simulink model "simulink_multirotor_v3_taimoor"  (R2021b)
settings: Solver=VariableStepAuto  StartTime=0.0  StopTime=10  RelTol=1e-3
libraries: slpidlib x6
settings Model: Creator=five  LastModifiedBy=Muham
settings SolverCC: AlgebraicLoopSolver=TrustRegion
settings DebuggingCC: SFMachineParentedDataDiag=warning

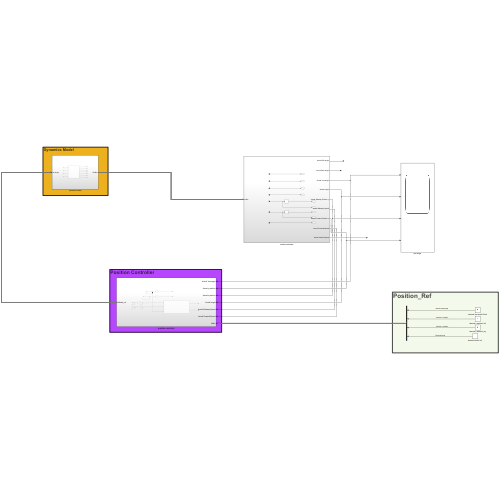
[thumbnail: Simulink's stored preview of the top-level diagram]
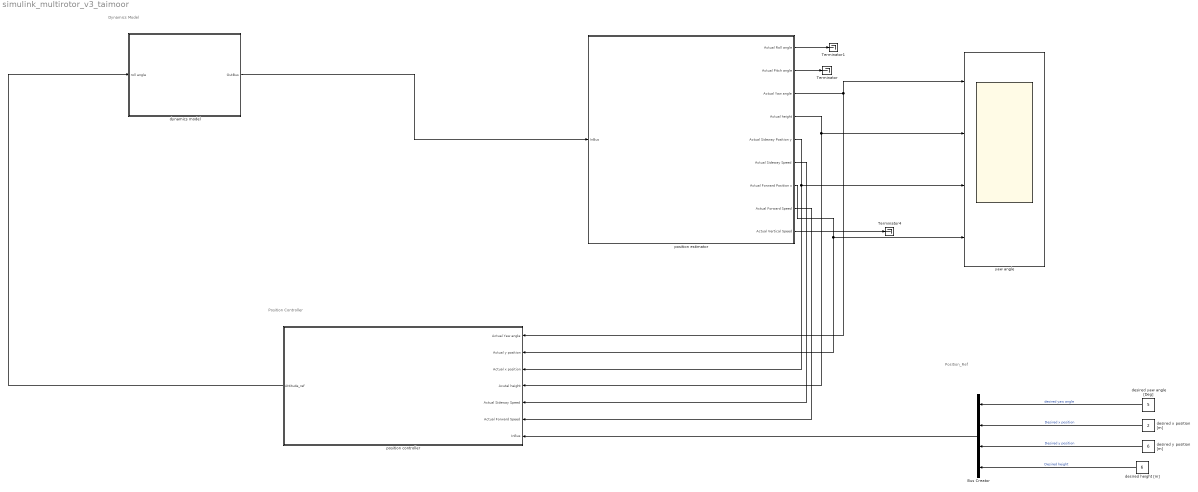
== system simulink_multirotor_v3_taimoor ==
  note: Dynamics Model
  note: Position Controller
  note: Position_Ref
  Bus Creator : BusCreator  Inputs=4
  Terminator : Terminator
  Terminator1 : Terminator
  Terminator4 : Terminator
  desired height [m] : Constant  Value=6
  desired x position [m] : Constant  Value=2
  desired y position [m] : Constant  Value=6
  desired yaw angle [Deg] : Constant  Value=5
  dynamics model : Subsystem
  position controller : Subsystem
  position estimator : Subsystem
  yaw angle : Scope  NumInputPorts=4
  wires:
  position estimator/4(Actual height) -> yaw angle/2, position controller/4(Acutal height)
  position estimator/7(Actual Forward Position x) -> position controller/2(Actual y position), yaw angle/4
  position estimator/5(Actual Sideway Position y) -> yaw angle/3, position controller/3(Actual x position)
  position estimator/3(Actual Yaw angle) -> yaw angle/1, position controller/1(Actual Yaw angle)
  position estimator/9(Actual Vertical Speed) -> Terminator4/1
  position estimator/8(Actual Forward Speed) -> position controller/6(Actual Forward Speed)
  position estimator/6(Actual Sideway Speed) -> position controller/5(Actual Sideway Speed)
  position estimator/2(Actual Pitch angle) -> Terminator/1
  position estimator/1(Actual Roll angle) -> Terminator1/1
  desired yaw angle [Deg]/1 -> Bus Creator/1  "desired yaw angle"
  desired x position [m]/1 -> Bus Creator/2  "Desired x position"
  desired y position [m]/1 -> Bus Creator/3  "Desired y position"
  desired height [m]/1 -> Bus Creator/4  "Desired height"
  Bus Creator/1 -> position controller/7(InBus)
  position controller/1(Attitude_ref) -> dynamics model/1(roll angle)
  dynamics model/1(OutBus) -> position estimator/1(InBus)

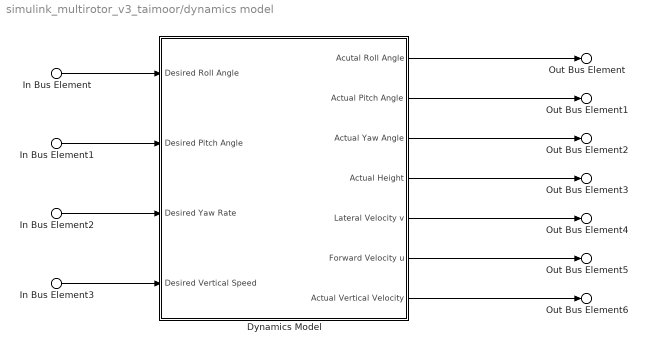
== system simulink_multirotor_v3_taimoor/dynamics model ==
  In Bus Element : Inport  PortName=roll angle  Element=desired roll angle
  In Bus Element1 : Inport  PortName=roll angle  Element=desired pitch angle
  In Bus Element2 : Inport  PortName=roll angle  Element=desired yaw rate
  In Bus Element3 : Inport  PortName=roll angle  Element=desired vertical speed
  Dynamics Model : Subsystem
  Out Bus Element : Outport  PortName=OutBus  Element=Actual Roll Angle
  Out Bus Element1 : Outport  PortName=OutBus  Element=Acutal Ptich Angle
  Out Bus Element2 : Outport  PortName=OutBus  Element=Actual Yaw Angle
  Out Bus Element3 : Outport  PortName=OutBus  Element=Actual Height
  Out Bus Element4 : Outport  PortName=OutBus  Element=Actual Sideway Speed
  Out Bus Element5 : Outport  PortName=OutBus  Element=Actual Forward Speed
  Out Bus Element6 : Outport  PortName=OutBus  Element=Actual Vertical Speed
  wires:
  In Bus Element/1 -> Dynamics Model/1(Desired Roll Angle)
  In Bus Element1/1 -> Dynamics Model/2(Desired Pitch Angle)
  In Bus Element2/1 -> Dynamics Model/3(Desired Yaw Rate)
  In Bus Element3/1 -> Dynamics Model/4(Desired Vertical Speed)
  Dynamics Model/6(Forward Velocity u) -> Out Bus Element5/1
  Dynamics Model/5(Lateral Velocity v) -> Out Bus Element4/1
  Dynamics Model/4(Actual Height) -> Out Bus Element3/1
  Dynamics Model/3(Actual Yaw Angle) -> Out Bus Element2/1
  Dynamics Model/2(Actual Pitch Angle) -> Out Bus Element1/1
  Dynamics Model/1(Acutal Roll Angle) -> Out Bus Element/1
  Dynamics Model/7(Actual Vertical Velocity) -> Out Bus Element6/1

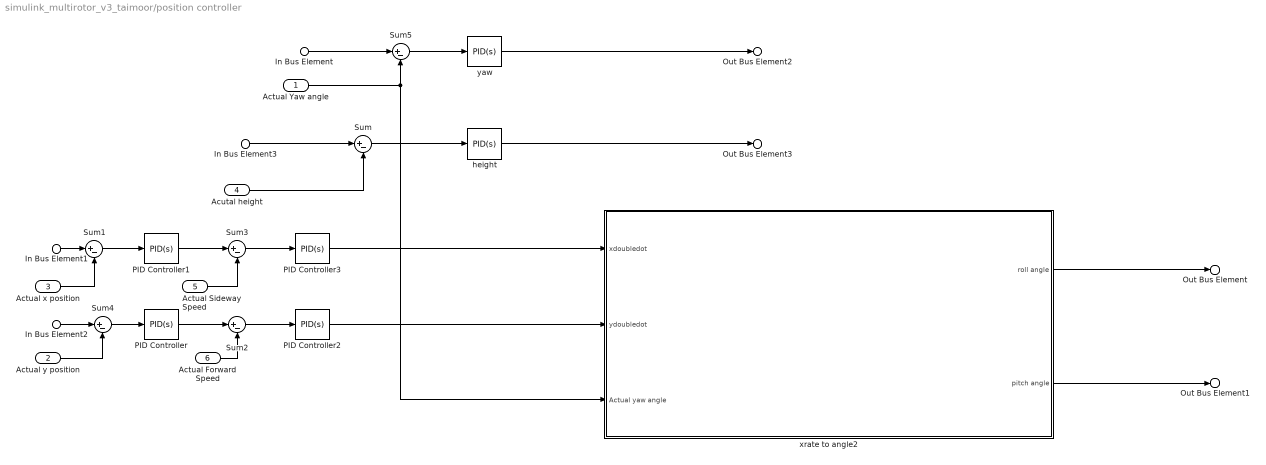
== system simulink_multirotor_v3_taimoor/position controller ==
  Actual Yaw angle : Inport
  Actual y position : Inport  Port=2
  Actual x position : Inport  Port=3
  Acutal height : Inport  Port=4
  Actual Sideway Speed : Inport  Port=5
  Actual Forward Speed : Inport  Port=6
  In Bus Element : Inport  Port=7  PortName=InBus  Element=desired yaw angle
  In Bus Element1 : Inport  Port=7  PortName=InBus  Element=Desired x position
  In Bus Element2 : Inport  Port=7  PortName=InBus  Element=Desired y position
  In Bus Element3 : Inport  Port=7  PortName=InBus  Element=Desired height
  PID Controller : slpidlib/PID Controller  Controller=PID  Form=Parallel  TimeDomain=Continuous-time  UseExternalTs=off  SampleTime=-1  IntegratorMethod=Forward Euler  FilterMethod=Forward Euler  ControllerParametersSource=internal  P=3  I=0  D=4  UseFilter=on  N=100  TunerSelectOption=Transfer Function Based (PID Tuner App)  InitialConditionSource=internal  InitialConditionForIntegrator=0  InitialConditionForFilter=0  DifferentiatorICPrevScaledInput=0  ExternalReset=none  TrackingMode=off  Kt=1  LimitOutput=off  SatLimitsSource=internal  UpperSaturationLimit=inf  LowerSaturationLimit=-inf  LinearizeAsGain=on  AntiWindupMode=none  Kb=1  POutMin=[]  POutMax=[]  IOutMin=[]  IOutMax=[]  DOutMin=[]  DOutMax=[]  NOutMin=[]  NOutMax=[]  SumOutMin=[]  SumOutMax=[]  SaturationOutMin=[]  SaturationOutMax=[]  PParamMin=[]  PParamMax=[]  IParamMin=[]  IParamMax=[]  DParamMin=[]  DParamMax=[]  NParamMin=[]  NParamMax=[]  KbParamMin=[]  KbParamMax=[]  KtParamMin=[]  KtParamMax=[]  KbOutMin=[]  KbOutMax=[]  KtOutMin=[]  KtOutMax=[]  IntegratorOutMin=[]  IntegratorOutMax=[]  FilterOutMin=[]  FilterOutMax=[]  SumI1OutMin=[]  SumI1OutMax=[]  SumI2OutMin=[]  SumI2OutMax=[]  SumI3OutMin=[]  SumI3OutMax=[]  SumI4OutMin=[]  SumI4OutMax=[]  SumDOutMin=[]  SumDOutMax=[]  DifferentiatorOutMin=[]  DifferentiatorOutMax=[]  FilterDiffOutCoefMin=[]  FilterDiffOutCoefMax=[]  ReciprocalOutMin=[]  ReciprocalOutMax=[]  SumDenOutMin=[]  SumDenOutMax=[]  SumNumOutMin=[]  SumNumOutMax=[]  DivideOutMin=[]  DivideOutMax=[]  UdiffTsProdOutMin=[]  UdiffTsProdOutMax=[]  NTsProdOutMin=[]  NTsProdOutMax=[]  UintegralTsProdOutMin=[]  UintegralTsProdOutMax=[]  UngainTsProdOutMin=[]  UngainTsProdOutMax=[]  IntegratorContinuousStateAttributes=''  IntegratorStateMustResolveToSignalObject=off  IntegratorRTWStateStorageClass=Auto  FilterContinuousStateAttributes=''  FilterStateMustResolveToSignalObject=off  FilterRTWStateStorageClass=Auto  ParallelPVariant=InternalParameters  IdealPVariant=Disabled  IVariant=InternalParameters  DVariant=InternalParameters  IntegratorVariant=Continuous  SatVariant=Disabled  AWVariant=Passthrough  PCopyVariant=Disabled  TRVariant=Disabled  FdbkBlocksVariant=Forward  IdealPFdbkVariant=Disabled  SatFdbkVariant=Disabled  DerivativeFilterVariant=ContFilter  NVariant=InternalParameters  NCopyVariant=Disabled  FilterICVariant=InternalICsFilter  IntegratorICVariant=InternalICs  ExternalResetVariant=Disabled  TRSumVariant=Passthrough  SumFdbkVariant=Disabled  SumVariant=Sum_PID  TsampFilterVariant=InternalTs  TsampNgainVariant=Passthrough  TsampIntegralVariant=Passthrough  ExternalSaturationOutDataTypeStr=Inherit: Same as second input
  PID Controller1 : slpidlib/PID Controller  Controller=PID  Form=Parallel  TimeDomain=Continuous-time  UseExternalTs=off  SampleTime=-1  IntegratorMethod=Forward Euler  FilterMethod=Forward Euler  ControllerParametersSource=internal  P=3  I=0  D=1  UseFilter=on  N=100  TunerSelectOption=Transfer Function Based (PID Tuner App)  InitialConditionSource=internal  InitialConditionForIntegrator=0  InitialConditionForFilter=0  DifferentiatorICPrevScaledInput=0  ExternalReset=none  TrackingMode=off  Kt=1  LimitOutput=off  SatLimitsSource=internal  UpperSaturationLimit=inf  LowerSaturationLimit=-inf  LinearizeAsGain=on  AntiWindupMode=none  Kb=1  POutMin=[]  POutMax=[]  IOutMin=[]  IOutMax=[]  DOutMin=[]  DOutMax=[]  NOutMin=[]  NOutMax=[]  SumOutMin=[]  SumOutMax=[]  SaturationOutMin=[]  SaturationOutMax=[]  PParamMin=[]  PParamMax=[]  IParamMin=[]  IParamMax=[]  DParamMin=[]  DParamMax=[]  NParamMin=[]  NParamMax=[]  KbParamMin=[]  KbParamMax=[]  KtParamMin=[]  KtParamMax=[]  KbOutMin=[]  KbOutMax=[]  KtOutMin=[]  KtOutMax=[]  IntegratorOutMin=[]  IntegratorOutMax=[]  FilterOutMin=[]  FilterOutMax=[]  SumI1OutMin=[]  SumI1OutMax=[]  SumI2OutMin=[]  SumI2OutMax=[]  SumI3OutMin=[]  SumI3OutMax=[]  SumI4OutMin=[]  SumI4OutMax=[]  SumDOutMin=[]  SumDOutMax=[]  DifferentiatorOutMin=[]  DifferentiatorOutMax=[]  FilterDiffOutCoefMin=[]  FilterDiffOutCoefMax=[]  ReciprocalOutMin=[]  ReciprocalOutMax=[]  SumDenOutMin=[]  SumDenOutMax=[]  SumNumOutMin=[]  SumNumOutMax=[]  DivideOutMin=[]  DivideOutMax=[]  UdiffTsProdOutMin=[]  UdiffTsProdOutMax=[]  NTsProdOutMin=[]  NTsProdOutMax=[]  UintegralTsProdOutMin=[]  UintegralTsProdOutMax=[]  UngainTsProdOutMin=[]  UngainTsProdOutMax=[]  IntegratorContinuousStateAttributes=''  IntegratorStateMustResolveToSignalObject=off  IntegratorRTWStateStorageClass=Auto  FilterContinuousStateAttributes=''  FilterStateMustResolveToSignalObject=off  FilterRTWStateStorageClass=Auto  ParallelPVariant=InternalParameters  IdealPVariant=Disabled  IVariant=InternalParameters  DVariant=InternalParameters  IntegratorVariant=Continuous  SatVariant=Disabled  AWVariant=Passthrough  PCopyVariant=Disabled  TRVariant=Disabled  FdbkBlocksVariant=Forward  IdealPFdbkVariant=Disabled  SatFdbkVariant=Disabled  DerivativeFilterVariant=ContFilter  NVariant=InternalParameters  NCopyVariant=Disabled  FilterICVariant=InternalICsFilter  IntegratorICVariant=InternalICs  ExternalResetVariant=Disabled  TRSumVariant=Passthrough  SumFdbkVariant=Disabled  SumVariant=Sum_PID  TsampFilterVariant=InternalTs  TsampNgainVariant=Passthrough  TsampIntegralVariant=Passthrough  ExternalSaturationOutDataTypeStr=Inherit: Same as second input
  PID Controller2 : slpidlib/PID Controller  Controller=PID  Form=Parallel  TimeDomain=Continuous-time  UseExternalTs=off  SampleTime=-1  IntegratorMethod=Forward Euler  FilterMethod=Forward Euler  ControllerParametersSource=internal  P=10  I=5  D=2.5  UseFilter=on  N=100  TunerSelectOption=Transfer Function Based (PID Tuner App)  InitialConditionSource=internal  InitialConditionForIntegrator=0  InitialConditionForFilter=0  DifferentiatorICPrevScaledInput=0  ExternalReset=none  TrackingMode=off  Kt=1  LimitOutput=off  SatLimitsSource=internal  UpperSaturationLimit=inf  LowerSaturationLimit=-inf  LinearizeAsGain=on  AntiWindupMode=none  Kb=1  POutMin=[]  POutMax=[]  IOutMin=[]  IOutMax=[]  DOutMin=[]  DOutMax=[]  NOutMin=[]  NOutMax=[]  SumOutMin=[]  SumOutMax=[]  SaturationOutMin=[]  SaturationOutMax=[]  PParamMin=[]  PParamMax=[]  IParamMin=[]  IParamMax=[]  DParamMin=[]  DParamMax=[]  NParamMin=[]  NParamMax=[]  KbParamMin=[]  KbParamMax=[]  KtParamMin=[]  KtParamMax=[]  KbOutMin=[]  KbOutMax=[]  KtOutMin=[]  KtOutMax=[]  IntegratorOutMin=[]  IntegratorOutMax=[]  FilterOutMin=[]  FilterOutMax=[]  SumI1OutMin=[]  SumI1OutMax=[]  SumI2OutMin=[]  SumI2OutMax=[]  SumI3OutMin=[]  SumI3OutMax=[]  SumI4OutMin=[]  SumI4OutMax=[]  SumDOutMin=[]  SumDOutMax=[]  DifferentiatorOutMin=[]  DifferentiatorOutMax=[]  FilterDiffOutCoefMin=[]  FilterDiffOutCoefMax=[]  ReciprocalOutMin=[]  ReciprocalOutMax=[]  SumDenOutMin=[]  SumDenOutMax=[]  SumNumOutMin=[]  SumNumOutMax=[]  DivideOutMin=[]  DivideOutMax=[]  UdiffTsProdOutMin=[]  UdiffTsProdOutMax=[]  NTsProdOutMin=[]  NTsProdOutMax=[]  UintegralTsProdOutMin=[]  UintegralTsProdOutMax=[]  UngainTsProdOutMin=[]  UngainTsProdOutMax=[]  IntegratorContinuousStateAttributes=''  IntegratorStateMustResolveToSignalObject=off  IntegratorRTWStateStorageClass=Auto  FilterContinuousStateAttributes=''  FilterStateMustResolveToSignalObject=off  FilterRTWStateStorageClass=Auto  ParallelPVariant=InternalParameters  IdealPVariant=Disabled  IVariant=InternalParameters  DVariant=InternalParameters  IntegratorVariant=Continuous  SatVariant=Disabled  AWVariant=Passthrough  PCopyVariant=Disabled  TRVariant=Disabled  FdbkBlocksVariant=Forward  IdealPFdbkVariant=Disabled  SatFdbkVariant=Disabled  DerivativeFilterVariant=ContFilter  NVariant=InternalParameters  NCopyVariant=Disabled  FilterICVariant=InternalICsFilter  IntegratorICVariant=InternalICs  ExternalResetVariant=Disabled  TRSumVariant=Passthrough  SumFdbkVariant=Disabled  SumVariant=Sum_PID  TsampFilterVariant=InternalTs  TsampNgainVariant=Passthrough  TsampIntegralVariant=Passthrough  ExternalSaturationOutDataTypeStr=Inherit: Same as second input
  PID Controller3 : slpidlib/PID Controller  Controller=PID  Form=Parallel  TimeDomain=Continuous-time  UseExternalTs=off  SampleTime=-1  IntegratorMethod=Forward Euler  FilterMethod=Forward Euler  ControllerParametersSource=internal  P=10  I=5  D=2.5  UseFilter=on  N=100  TunerSelectOption=Transfer Function Based (PID Tuner App)  InitialConditionSource=internal  InitialConditionForIntegrator=0  InitialConditionForFilter=0  DifferentiatorICPrevScaledInput=0  ExternalReset=none  TrackingMode=off  Kt=1  LimitOutput=off  SatLimitsSource=internal  UpperSaturationLimit=inf  LowerSaturationLimit=-inf  LinearizeAsGain=on  AntiWindupMode=none  Kb=1  POutMin=[]  POutMax=[]  IOutMin=[]  IOutMax=[]  DOutMin=[]  DOutMax=[]  NOutMin=[]  NOutMax=[]  SumOutMin=[]  SumOutMax=[]  SaturationOutMin=[]  SaturationOutMax=[]  PParamMin=[]  PParamMax=[]  IParamMin=[]  IParamMax=[]  DParamMin=[]  DParamMax=[]  NParamMin=[]  NParamMax=[]  KbParamMin=[]  KbParamMax=[]  KtParamMin=[]  KtParamMax=[]  KbOutMin=[]  KbOutMax=[]  KtOutMin=[]  KtOutMax=[]  IntegratorOutMin=[]  IntegratorOutMax=[]  FilterOutMin=[]  FilterOutMax=[]  SumI1OutMin=[]  SumI1OutMax=[]  SumI2OutMin=[]  SumI2OutMax=[]  SumI3OutMin=[]  SumI3OutMax=[]  SumI4OutMin=[]  SumI4OutMax=[]  SumDOutMin=[]  SumDOutMax=[]  DifferentiatorOutMin=[]  DifferentiatorOutMax=[]  FilterDiffOutCoefMin=[]  FilterDiffOutCoefMax=[]  ReciprocalOutMin=[]  ReciprocalOutMax=[]  SumDenOutMin=[]  SumDenOutMax=[]  SumNumOutMin=[]  SumNumOutMax=[]  DivideOutMin=[]  DivideOutMax=[]  UdiffTsProdOutMin=[]  UdiffTsProdOutMax=[]  NTsProdOutMin=[]  NTsProdOutMax=[]  UintegralTsProdOutMin=[]  UintegralTsProdOutMax=[]  UngainTsProdOutMin=[]  UngainTsProdOutMax=[]  IntegratorContinuousStateAttributes=''  IntegratorStateMustResolveToSignalObject=off  IntegratorRTWStateStorageClass=Auto  FilterContinuousStateAttributes=''  FilterStateMustResolveToSignalObject=off  FilterRTWStateStorageClass=Auto  ParallelPVariant=InternalParameters  IdealPVariant=Disabled  IVariant=InternalParameters  DVariant=InternalParameters  IntegratorVariant=Continuous  SatVariant=Disabled  AWVariant=Passthrough  PCopyVariant=Disabled  TRVariant=Disabled  FdbkBlocksVariant=Forward  IdealPFdbkVariant=Disabled  SatFdbkVariant=Disabled  DerivativeFilterVariant=ContFilter  NVariant=InternalParameters  NCopyVariant=Disabled  FilterICVariant=InternalICsFilter  IntegratorICVariant=InternalICs  ExternalResetVariant=Disabled  TRSumVariant=Passthrough  SumFdbkVariant=Disabled  SumVariant=Sum_PID  TsampFilterVariant=InternalTs  TsampNgainVariant=Passthrough  TsampIntegralVariant=Passthrough  ExternalSaturationOutDataTypeStr=Inherit: Same as second input
  Sum{,1..5} (6 alike) : Sum  Inputs=|+-
  height : slpidlib/PID Controller  Controller=PID  Form=Parallel  TimeDomain=Continuous-time  UseExternalTs=off  SampleTime=-1  IntegratorMethod=Forward Euler  FilterMethod=Forward Euler  ControllerParametersSource=internal  P=1  I=0  D=4  UseFilter=on  N=100  TunerSelectOption=Transfer Function Based (PID Tuner App)  InitialConditionSource=internal  InitialConditionForIntegrator=0  InitialConditionForFilter=0  DifferentiatorICPrevScaledInput=0  ExternalReset=none  TrackingMode=off  Kt=1  LimitOutput=off  SatLimitsSource=internal  UpperSaturationLimit=inf  LowerSaturationLimit=-inf  LinearizeAsGain=on  AntiWindupMode=none  Kb=1  POutMin=[]  POutMax=[]  IOutMin=[]  IOutMax=[]  DOutMin=[]  DOutMax=[]  NOutMin=[]  NOutMax=[]  SumOutMin=[]  SumOutMax=[]  SaturationOutMin=[]  SaturationOutMax=[]  PParamMin=[]  PParamMax=[]  IParamMin=[]  IParamMax=[]  DParamMin=[]  DParamMax=[]  NParamMin=[]  NParamMax=[]  KbParamMin=[]  KbParamMax=[]  KtParamMin=[]  KtParamMax=[]  KbOutMin=[]  KbOutMax=[]  KtOutMin=[]  KtOutMax=[]  IntegratorOutMin=[]  IntegratorOutMax=[]  FilterOutMin=[]  FilterOutMax=[]  SumI1OutMin=[]  SumI1OutMax=[]  SumI2OutMin=[]  SumI2OutMax=[]  SumI3OutMin=[]  SumI3OutMax=[]  SumI4OutMin=[]  SumI4OutMax=[]  SumDOutMin=[]  SumDOutMax=[]  DifferentiatorOutMin=[]  DifferentiatorOutMax=[]  FilterDiffOutCoefMin=[]  FilterDiffOutCoefMax=[]  ReciprocalOutMin=[]  ReciprocalOutMax=[]  SumDenOutMin=[]  SumDenOutMax=[]  SumNumOutMin=[]  SumNumOutMax=[]  DivideOutMin=[]  DivideOutMax=[]  UdiffTsProdOutMin=[]  UdiffTsProdOutMax=[]  NTsProdOutMin=[]  NTsProdOutMax=[]  UintegralTsProdOutMin=[]  UintegralTsProdOutMax=[]  UngainTsProdOutMin=[]  UngainTsProdOutMax=[]  IntegratorContinuousStateAttributes=''  IntegratorStateMustResolveToSignalObject=off  IntegratorRTWStateStorageClass=Auto  FilterContinuousStateAttributes=''  FilterStateMustResolveToSignalObject=off  FilterRTWStateStorageClass=Auto  ParallelPVariant=InternalParameters  IdealPVariant=Disabled  IVariant=InternalParameters  DVariant=InternalParameters  IntegratorVariant=Continuous  SatVariant=Disabled  AWVariant=Passthrough  PCopyVariant=Disabled  TRVariant=Disabled  FdbkBlocksVariant=Forward  IdealPFdbkVariant=Disabled  SatFdbkVariant=Disabled  DerivativeFilterVariant=ContFilter  NVariant=InternalParameters  NCopyVariant=Disabled  FilterICVariant=InternalICsFilter  IntegratorICVariant=InternalICs  ExternalResetVariant=Disabled  TRSumVariant=Passthrough  SumFdbkVariant=Disabled  SumVariant=Sum_PID  TsampFilterVariant=InternalTs  TsampNgainVariant=Passthrough  TsampIntegralVariant=Passthrough  ExternalSaturationOutDataTypeStr=Inherit: Same as second input
  xrate to angle2 : Subsystem
  yaw : slpidlib/PID Controller  Controller=PID  Form=Parallel  TimeDomain=Continuous-time  UseExternalTs=off  SampleTime=-1  IntegratorMethod=Forward Euler  FilterMethod=Forward Euler  ControllerParametersSource=internal  P=50  I=10  D=2.5  UseFilter=on  N=100  TunerSelectOption=Transfer Function Based (PID Tuner App)  InitialConditionSource=internal  InitialConditionForIntegrator=0  InitialConditionForFilter=0  DifferentiatorICPrevScaledInput=0  ExternalReset=none  TrackingMode=off  Kt=1  LimitOutput=off  SatLimitsSource=internal  UpperSaturationLimit=inf  LowerSaturationLimit=-inf  LinearizeAsGain=on  AntiWindupMode=none  Kb=1  POutMin=[]  POutMax=[]  IOutMin=[]  IOutMax=[]  DOutMin=[]  DOutMax=[]  NOutMin=[]  NOutMax=[]  SumOutMin=[]  SumOutMax=[]  SaturationOutMin=[]  SaturationOutMax=[]  PParamMin=[]  PParamMax=[]  IParamMin=[]  IParamMax=[]  DParamMin=[]  DParamMax=[]  NParamMin=[]  NParamMax=[]  KbParamMin=[]  KbParamMax=[]  KtParamMin=[]  KtParamMax=[]  KbOutMin=[]  KbOutMax=[]  KtOutMin=[]  KtOutMax=[]  IntegratorOutMin=[]  IntegratorOutMax=[]  FilterOutMin=[]  FilterOutMax=[]  SumI1OutMin=[]  SumI1OutMax=[]  SumI2OutMin=[]  SumI2OutMax=[]  SumI3OutMin=[]  SumI3OutMax=[]  SumI4OutMin=[]  SumI4OutMax=[]  SumDOutMin=[]  SumDOutMax=[]  DifferentiatorOutMin=[]  DifferentiatorOutMax=[]  FilterDiffOutCoefMin=[]  FilterDiffOutCoefMax=[]  ReciprocalOutMin=[]  ReciprocalOutMax=[]  SumDenOutMin=[]  SumDenOutMax=[]  SumNumOutMin=[]  SumNumOutMax=[]  DivideOutMin=[]  DivideOutMax=[]  UdiffTsProdOutMin=[]  UdiffTsProdOutMax=[]  NTsProdOutMin=[]  NTsProdOutMax=[]  UintegralTsProdOutMin=[]  UintegralTsProdOutMax=[]  UngainTsProdOutMin=[]  UngainTsProdOutMax=[]  IntegratorContinuousStateAttributes=''  IntegratorStateMustResolveToSignalObject=off  IntegratorRTWStateStorageClass=Auto  FilterContinuousStateAttributes=''  FilterStateMustResolveToSignalObject=off  FilterRTWStateStorageClass=Auto  ParallelPVariant=InternalParameters  IdealPVariant=Disabled  IVariant=InternalParameters  DVariant=InternalParameters  IntegratorVariant=Continuous  SatVariant=Disabled  AWVariant=Passthrough  PCopyVariant=Disabled  TRVariant=Disabled  FdbkBlocksVariant=Forward  IdealPFdbkVariant=Disabled  SatFdbkVariant=Disabled  DerivativeFilterVariant=ContFilter  NVariant=InternalParameters  NCopyVariant=Disabled  FilterICVariant=InternalICsFilter  IntegratorICVariant=InternalICs  ExternalResetVariant=Disabled  TRSumVariant=Passthrough  SumFdbkVariant=Disabled  SumVariant=Sum_PID  TsampFilterVariant=InternalTs  TsampNgainVariant=Passthrough  TsampIntegralVariant=Passthrough  ExternalSaturationOutDataTypeStr=Inherit: Same as second input
  Out Bus Element : Outport  PortName=Attitude_ref  Element=desired roll angle
  Out Bus Element1 : Outport  PortName=Attitude_ref  Element=desired pitch angle
  Out Bus Element2 : Outport  PortName=Attitude_ref  Element=desired yaw rate
  Out Bus Element3 : Outport  PortName=Attitude_ref  Element=desired vertical speed
  wires:
  In Bus Element/1 -> Sum5/1
  Actual Yaw angle/1 -> Sum5/2, xrate to angle2/3(Actual yaw angle)
  Acutal height/1 -> Sum/2
  In Bus Element3/1 -> Sum/1
  In Bus Element1/1 -> Sum1/1
  Actual x position/1 -> Sum1/2
  In Bus Element2/1 -> Sum4/1
  Actual y position/1 -> Sum4/2
  Sum/1 -> height/1
  Sum5/1 -> yaw/1
  Sum4/1 -> PID Controller/1
  PID Controller/1 -> Sum2/1
  Sum1/1 -> PID Controller1/1
  PID Controller1/1 -> Sum3/1
  Actual Sideway Speed/1 -> Sum3/2
  Actual Forward Speed/1 -> Sum2/2
  Sum2/1 -> PID Controller2/1
  Sum3/1 -> PID Controller3/1
  xrate to angle2/2(pitch angle) -> Out Bus Element1/1
  xrate to angle2/1(roll angle) -> Out Bus Element/1
  height/1 -> Out Bus Element3/1
  yaw/1 -> Out Bus Element2/1
  PID Controller3/1 -> xrate to angle2/1(xdoubledot)
  PID Controller2/1 -> xrate to angle2/2(ydoubledot)

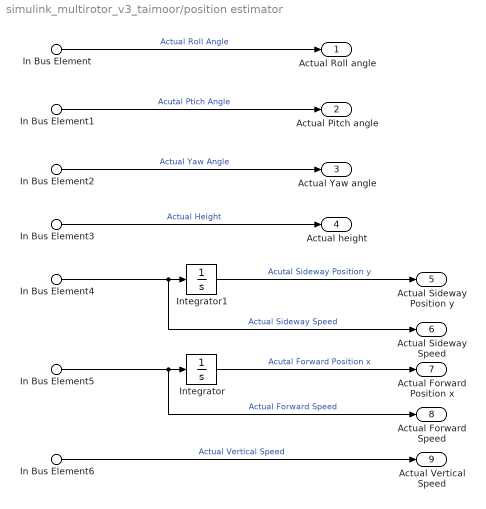
== system simulink_multirotor_v3_taimoor/position estimator ==
  In Bus Element : Inport  PortName=InBus  Element=Actual Roll Angle
  In Bus Element1 : Inport  PortName=InBus  Element=Acutal Ptich Angle
  In Bus Element2 : Inport  PortName=InBus  Element=Actual Yaw Angle
  In Bus Element3 : Inport  PortName=InBus  Element=Actual Height
  In Bus Element4 : Inport  PortName=InBus  Element=Actual Sideway Speed
  In Bus Element5 : Inport  PortName=InBus  Element=Actual Forward Speed
  In Bus Element6 : Inport  PortName=InBus  Element=Actual Vertical Speed
  Integrator : Integrator
  Integrator1 : Integrator
  Actual Roll angle : Outport
  Actual Pitch angle : Outport  Port=2
  Actual Yaw angle : Outport  Port=3
  Actual height : Outport  Port=4
  Actual Sideway Position y : Outport  Port=5
  Actual Sideway Speed : Outport  Port=6
  Actual Forward Position x : Outport  Port=7
  Actual Forward Speed : Outport  Port=8
  Actual Vertical Speed : Outport  Port=9
  wires:
  In Bus Element5/1 -> Actual Forward Speed/1, Integrator/1  "Actual Forward Speed"
  In Bus Element2/1 -> Actual Yaw angle/1  "Actual Yaw Angle"
  In Bus Element6/1 -> Actual Vertical Speed/1  "Actual Vertical Speed"
  In Bus Element/1 -> Actual Roll angle/1  "Actual Roll Angle"
  Integrator/1 -> Actual Forward Position x/1  "Acutal Forward Position x"
  In Bus Element1/1 -> Actual Pitch angle/1  "Acutal Ptich Angle"
  In Bus Element3/1 -> Actual height/1  "Actual Height"
  In Bus Element4/1 -> Actual Sideway Speed/1, Integrator1/1  "Actual Sideway Speed"
  Integrator1/1 -> Actual Sideway Position y/1  "Acutal Sideway Position y"

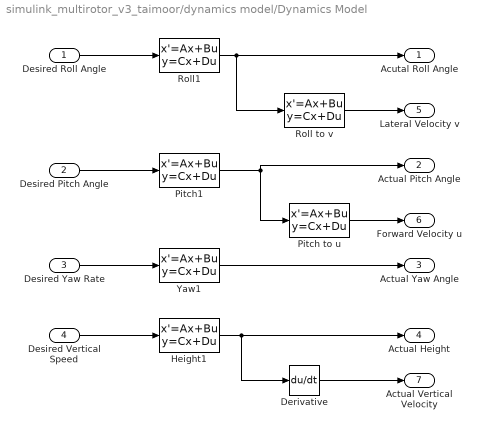
== system simulink_multirotor_v3_taimoor/dynamics model/Dynamics Model ==
  Desired Roll Angle : Inport
  Desired Pitch Angle : Inport  Port=2
  Desired Yaw Rate : Inport  Port=3
  Desired Vertical Speed : Inport  Port=4
  Derivative : Derivative
  Height1 : StateSpace  A=[-5.82 -3.6046e-6; 3.8147e-6 0]  B=[1024;0]  C=[1.4907e-4 1.3191e3]  D=0  InitialCondition=0
  Pitch to u : StateSpace  A=[-0.665]  B=[2]  C=[-3.0772]  D=0  InitialCondition=0
  Pitch1 : StateSpace  A=[-3.9784 -2.9796; 4 0]  B=[2;0]  C=[1.2569 0.6083]  D=0  InitialCondition=0
  Roll to v : StateSpace  A=[-0.4596]  B=[2]  C=[2.3868]  D=0  InitialCondition=0
  Roll1 : StateSpace  A=[-4.2683 -3.1716; 4 0]  B=[2;0]  C=[0.7417 0.4405]  D=0  InitialCondition=0
  Yaw1 : StateSpace  A=[-0.0059]  B=[1]  C=[1.2653]  D=0  InitialCondition=0
  Acutal Roll Angle : Outport
  Actual Pitch Angle : Outport  Port=2
  Actual Yaw Angle : Outport  Port=3
  Actual Height : Outport  Port=4
  Lateral Velocity v : Outport  Port=5
  Forward Velocity u : Outport  Port=6
  Actual Vertical Velocity : Outport  Port=7
  wires:
  Height1/1 -> Derivative/1, Actual Height/1
  Roll to v/1 -> Lateral Velocity v/1
  Yaw1/1 -> Actual Yaw Angle/1
  Pitch to u/1 -> Forward Velocity u/1
  Desired Yaw Rate/1 -> Yaw1/1
  Desired Roll Angle/1 -> Roll1/1
  Derivative/1 -> Actual Vertical Velocity/1
  Roll1/1 -> Roll to v/1, Acutal Roll Angle/1
  Desired Vertical Speed/1 -> Height1/1
  Pitch1/1 -> Pitch to u/1, Actual Pitch Angle/1
  Desired Pitch Angle/1 -> Pitch1/1

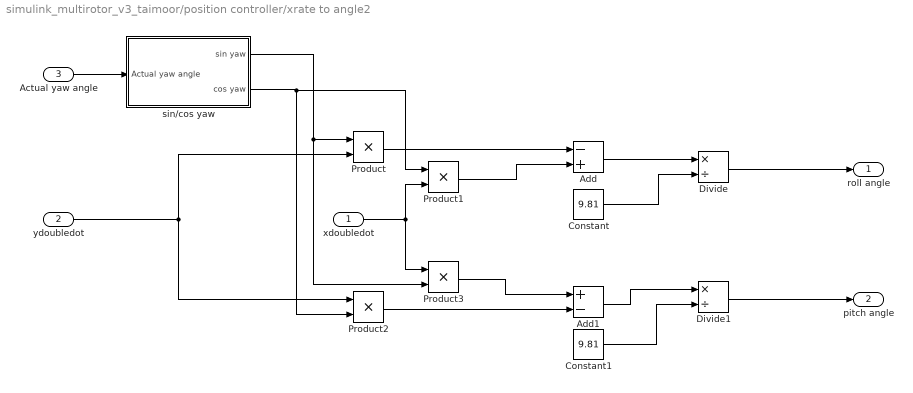
== system simulink_multirotor_v3_taimoor/position controller/xrate to angle2 ==
  xdoubledot : Inport
  ydoubledot : Inport  Port=2
  Actual yaw angle : Inport  Port=3
  Add : Sum  Inputs=-+
  Add1 : Sum  Inputs=+-
  Constant : Constant  Value=9.81
  Constant1 : Constant  Value=9.81
  Divide : Product  Inputs=*/
  Divide1 : Product  Inputs=*/
  Product{,1..3} (4 alike) : Product
  sin/cos yaw : Subsystem
  roll angle : Outport
  pitch angle : Outport  Port=2
  wires:
  Actual yaw angle/1 -> sin/cos yaw/1(Actual yaw angle)
  ydoubledot/1 -> Product/2, Product2/1
  Product/1 -> Add/1
  Product1/1 -> Add/2
  sin/cos yaw/2(cos yaw) -> Product2/2, Product1/1
  xdoubledot/1 -> Product1/2, Product3/1
  sin/cos yaw/1(sin yaw) -> Product3/2, Product/1
  Product2/1 -> Add1/2
  Product3/1 -> Add1/1
  Add1/1 -> Divide1/1
  Constant/1 -> Divide/2
  Add/1 -> Divide/1
  Divide/1 -> roll angle/1
  Divide1/1 -> pitch angle/1
  Constant1/1 -> Divide1/2

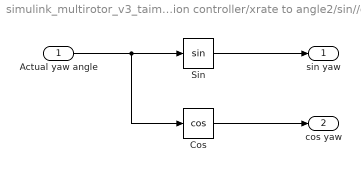
== system simulink_multirotor_v3_taimoor/position controller/xrate to angle2/sin//cos yaw ==
  Actual yaw angle : Inport
  Cos : Trigonometry  Operator=cos
  Sin : Trigonometry
  sin yaw : Outport
  cos yaw : Outport  Port=2
  wires:
  Actual yaw angle/1 -> Cos/1, Sin/1
  Sin/1 -> sin yaw/1
  Cos/1 -> cos yaw/1
